simulink model "symulacja_szumy"  (R2016a)
settings: Solver=ode5  StartTime=0.0  StopTime=150  FixedStep=0.01  RelTol=1e-3
values from neighbouring files (symbols this model uses):
  DEN = zeros(length(h_n), 6)    [model_strejc2.m]    (also in uruchom_symulacja_szumy.m = sym2poly((s+1)*(2*s+1)*(3*s+1)*(4*s+1)*(5*s+1)*(6*s+1)))
  NUM = 1    [model_strejc2.m]    (also in uruchom_symulacja_szumy.m)
libraries: simulink x1
settings Model: Creator=Kuba  LastModifiedBy=Kuba

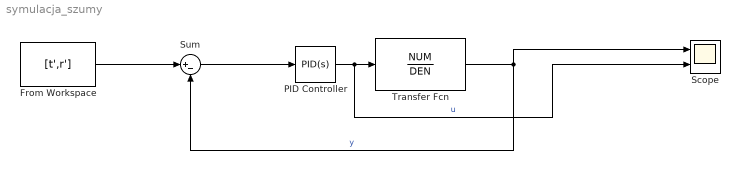
== system symulacja_szumy ==
  From Workspace : FromWorkspace  VariableName=[t',r']  SampleTime=0
  PID Controller : simulink/Continuous/PID Controller  Controller=PID  TimeDomain=Continuous-time  SampleTime=-1  IntegratorMethod=Forward Euler  FilterMethod=Forward Euler  Form=Parallel  UseFilter=on  ControllerParametersSource=internal  P=1.55873027592635  I=0.0949734870546304  D=6.21308599196381  N=12.2026128486554  InitialConditionSource=internal  InitialConditionForIntegrator=0  InitialConditionForFilter=0  ExternalReset=none  LimitOutput=off  UpperSaturationLimit=inf  LowerSaturationLimit=-inf  LinearizeAsGain=on  AntiWindupMode=none  Kb=1  TrackingMode=off  Kt=1  PParamMin=[]  PParamMax=[]  IParamMin=[]  IParamMax=[]  DParamMin=[]  DParamMax=[]  NParamMin=[]  NParamMax=[]  KbParamMin=[]  KbParamMax=[]  KtParamMin=[]  KtParamMax=[]  POutMin=[]  POutMax=[]  IOutMin=[]  IOutMax=[]  DOutMin=[]  DOutMax=[]  NOutMin=[]  NOutMax=[]  KbOutMin=[]  KbOutMax=[]  KtOutMin=[]  KtOutMax=[]  IntegratorOutMin=[]  IntegratorOutMax=[]  FilterOutMin=[]  FilterOutMax=[]  SumOutMin=[]  SumOutMax=[]  SumI1OutMin=[]  SumI1OutMax=[]  SumI2OutMin=[]  SumI2OutMax=[]  SumI3OutMin=[]  SumI3OutMax=[]  SumDOutMin=[]  SumDOutMax=[]  SaturationOutMin=[]  SaturationOutMax=[]  IntegratorContinuousStateAttributes=''  IntegratorStateMustResolveToSignalObject=off  IntegratorRTWStateStorageClass=Auto  FilterContinuousStateAttributes=''  FilterStateMustResolveToSignalObject=off  FilterRTWStateStorageClass=Auto  DifferentiatorICPrevScaledInput=0  DifferentiatorOutMin=[]  DifferentiatorOutMax=[]
  Scope : Scope  NumInputPorts=2
  Sum : Sum  Inputs=|+-
  Transfer Fcn : TransferFcn  Numerator=NUM  Denominator=DEN
  wires:
  From Workspace/1 -> Sum/1
  Sum/1 -> PID Controller/1
  PID Controller/1 -> Scope/2, Transfer Fcn/1  "u"
  Transfer Fcn/1 -> Scope/1, Sum/2  "y"
